simulink model "trackOnly"  (R2014a)
settings: Solver=FixedStepDiscrete  StartTime=0.0  StopTime=10.0  RelTol=1e-3
undefined symbols (not defined in the file or in its folder): fdesignblkfcn, gcbh
libraries: simulink x8, visionstatistics x5, visiontextngfix x2, embdlinuxlib x2
settings Model: SimulationMode=external  ExtModeTrigDuration=100  Creator=jsustare  LastModifiedBy=jsustare
settings OptimizationCC: OptimizeModelRefInitCode=on  LifeSpan=1
settings DebuggingCC: UnderspecifiedInitializationDetection=Classic  SolverPrmCheckMsg=none
settings HardwareCC: ProdLargestAtomicInteger=Long  ProdLargestAtomicFloat=Double  ProdEndianess=LittleEndian  ProdHWDeviceType=ARM Compatible->ARM Cortex
settings RTWCC: SystemTargetFile=realtime.tlc  GenerateMakefile=off  TemplateMakefile=realtime.tmf  Description=Run on Target Hardware  RTWVerbose=off  ProcessScript=realtime_make_rtw_hook
settings STFCustomTargetCC: TargetLibSuffix=.a  GenerateSampleERTMain=on  ConcurrentExecutionCompliant=off  GeneratePreprocessorConditionals=Use local settings  ERTCustomFileBanners=on  SupportNonInlinedSFcns=off  SupportVariableSizeSignals=on  MATLABClassNameForMDSCustomization=Simulink.SoftwareTarget.ERTCustomization  GRTInterface=off  SystemTargetFile=realtime.tlc
settings ERTTargetCC: CombineOutputUpdateFcns=off  SupportContinuousTime=on  SupportVariableSizeSignals=on  ExtModeMexArgs='169.254.0.31' 0 17725  ERTSrcFileBannerTemplate=realtime_code_template.cgt  ERTHdrFileBannerTemplate=realtime_code_template.cgt  ERTDataSrcFileTemplate=realtime_code_template.cgt  ERTDataHdrFileTemplate=realtime_code_template.cgt  ERTCustomFileTemplate=realtime_file_process.tlc

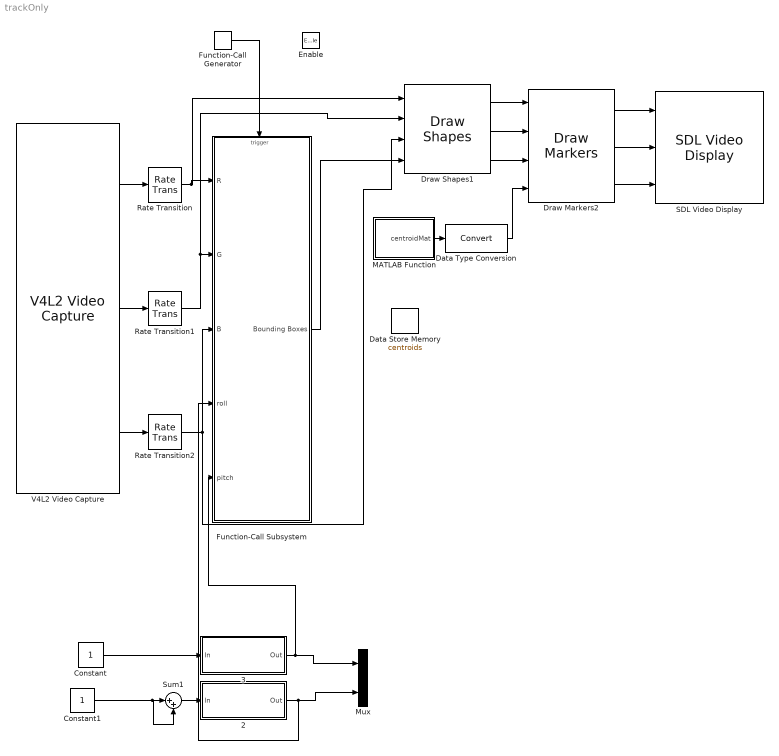
== system trackOnly ==
  Enable : EnablePort  PropagateVarSize=During execution
  " 2" : Subsystem  DialogController=fdesignblkfcn  InitFcn=fdesignblkfcn(gcbh, {'InitFcn'});  mask(Lowpass Filter){}
      mask help: Design a lowpass filter
      settings: CopyFcn=fdesignblkfcn(gcbh, {'CopyFcn'});
      mask Help: helpview(mapfilelocation('dsp'), 'dsplowpassfilter');
      mask Display: disp('Lowpass')
  " 3" : Subsystem  DialogController=fdesignblkfcn  InitFcn=fdesignblkfcn(gcbh, {'InitFcn'});  mask(Lowpass Filter){}
      mask help: Design a lowpass filter
      settings: CopyFcn=fdesignblkfcn(gcbh, {'CopyFcn'});
      mask Help: helpview(mapfilelocation('dsp'), 'dsplowpassfilter');
      mask Display: disp('Lowpass')
  Constant : Constant
  Constant1 : Constant
  Data Store Memory : DataStoreMemory  DataStoreName=centroids  ReadBeforeWriteMsg=warning  WriteAfterWriteMsg=warning  WriteAfterReadMsg=warning  InitialValue=zeros(13,2,4)  OutDataTypeStr=double
  Data Type Conversion : DataTypeConversion
  Draw Markers2 : visiontextngfix/Draw Markers  shape=X-mark  size=3  fill=off  fillClrSource=Specify via dialog  display=User-specified value  intensity=200  color=[255 255 255]  opacity=0.6  viewport=Entire image  antialiasing=off  inType=Obsolete  imagePorts=Separate color signals  prodOutputMode=Binary point scaling  prodOutputWordLength=32  prodOutputFracLength=14  memoryMode=Specify word length  memoryWordLength=16  memoryFracLength=15  roundingMode=Floor  overflowMode=off
  Draw Shapes1 : visiontextngfix/Draw Shapes  shape=Rectangles  fill=off  lineWidth=1  fillClrSource=Specify via dialog  display=User-specified value  intensity=200  color=[255 0 0]  opacity=0.6  viewport=Entire image  antialiasing=off  inType=Obsolete  imagePorts=Separate color signals  prodOutputMode=Binary point scaling  prodOutputWordLength=32  prodOutputFracLength=14  memoryMode=Specify word length  memoryWordLength=16  memoryFracLength=15  roundingMode=Floor  overflowMode=off
  Function-Call Generator : simulink/Ports & Subsystems/Function-Call Generator  sample_time=0.06  numberOfIterations=1
  Function-Call Subsystem : Subsystem  TreatAsAtomicUnit=on
  MATLAB Function : MATLAB Function  TreatAsAtomicUnit=on
  Mux : Mux  Inputs=2
  Rate Transition : RateTransition  Deterministic=off
  Rate Transition1 : RateTransition  Deterministic=off
  Rate Transition2 : RateTransition  Deterministic=off
  SDL Video Display : embdlinuxlib/SDL Video Display  pixelFormat=RGB  pixelOrder=Planar  rowMajor=on  blockPlatform=Raspberry Pi
  Sum1 : Sum  Inputs=|++
  V4L2 Video Capture : embdlinuxlib/V4L2 Video Capture  m_devName='/dev/video0'  roi=[0, 0, 640, 480]  imSizeSelection=320x240  imSize=[640, 480]  pixelFormat=RGB  pixelOrder=Planar  sampleTime=0.06  simOutput=Colorbars  blockPlatform=Raspberry Pi
  wires:
  V4L2 Video Capture/3 -> Rate Transition2/1
  V4L2 Video Capture/1 -> Rate Transition/1
  V4L2 Video Capture/2 -> Rate Transition1/1
  Function-Call Generator/1 -> Function-Call Subsystem/Trigger
  Function-Call Subsystem/1("Bounding Boxes ") -> Draw Shapes1/4
  Rate Transition/1 -> Draw Shapes1/1, Function-Call Subsystem/1(R)
  Rate Transition1/1 -> Draw Shapes1/2, Function-Call Subsystem/2(G)
  Rate Transition2/1 -> Draw Shapes1/3, Function-Call Subsystem/3(B)
  Data Type Conversion/1 -> Draw Markers2/4
  Draw Markers2/2 -> SDL Video Display/2
  Draw Markers2/3 -> SDL Video Display/3
  Draw Markers2/1 -> SDL Video Display/1
  Draw Shapes1/3 -> Draw Markers2/3
  Draw Shapes1/2 -> Draw Markers2/2
  Draw Shapes1/1 -> Draw Markers2/1
  " 2"/1(Out) -> Function-Call Subsystem/4(roll), Mux/2
  " 3"/1(Out) -> Function-Call Subsystem/5(pitch), Mux/1
  Sum1/1 -> " 2"/1(In)
  MATLAB Function/1(centroidMat) -> Data Type Conversion/1
  Constant/1 -> " 3"/1(In)
  Constant1/1 -> Sum1/2, Sum1/1

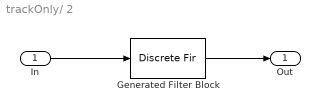
== system trackOnly/ 2 ==
  In : Inport
  Generated Filter Block : DiscreteFir  Tag=BlockMethodSubSystem  Coefficients=[0.0032276888738420255 -0.012093185057654832 -0.056871256727662273 -0.033025317279675399 0.16717851315296134 0.40566714821275895 0.40566714821275895 0.16717851315296134 -0.033025317279675399 -0.056871256727662273 -0.012093185057654832 0.0032276888738420255]  InputProcessing=Columns as channels (frame based)
  Out : Outport
  wires:
  Generated Filter Block/1 -> Out/1
  In/1 -> Generated Filter Block/1

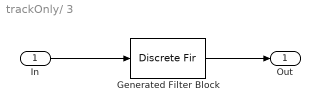
== system trackOnly/ 3 ==
  In : Inport
  Generated Filter Block : DiscreteFir  Tag=BlockMethodSubSystem  Coefficients=[0.0032276888738420255 -0.012093185057654832 -0.056871256727662273 -0.033025317279675399 0.16717851315296134 0.40566714821275895 0.40566714821275895 0.16717851315296134 -0.033025317279675399 -0.056871256727662273 -0.012093185057654832 0.0032276888738420255]  InputProcessing=Columns as channels (frame based)
  Out : Outport
  wires:
  In/1 -> Generated Filter Block/1
  Generated Filter Block/1 -> Out/1

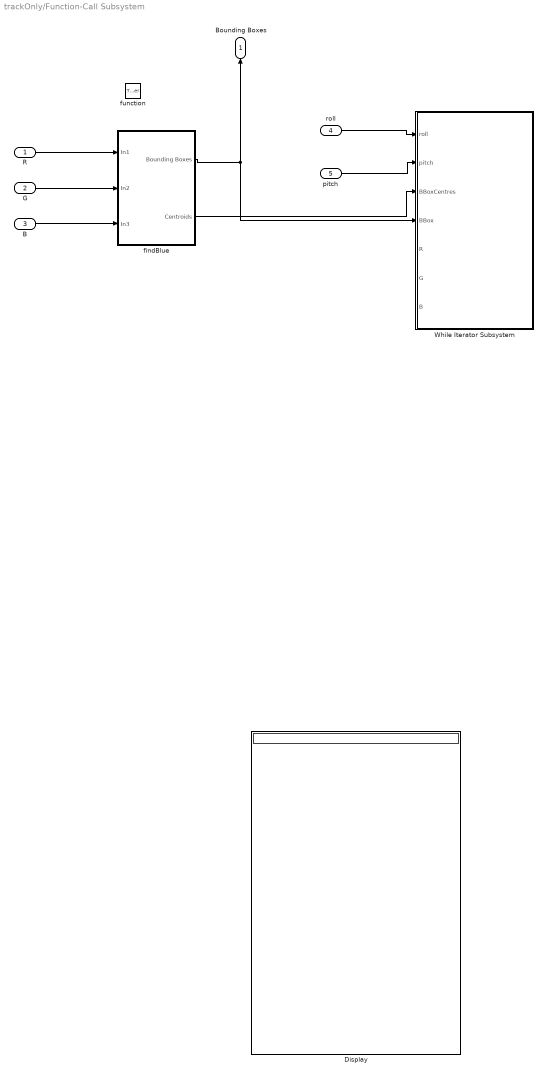
== system trackOnly/Function-Call Subsystem ==
  R : Inport
  G : Inport  Port=2
  B : Inport  Port=3
  roll : Inport  Port=4
  pitch : Inport  Port=5
  function : TriggerPort  TriggerType=function-call
  Display : Display
  While Iterator Subsystem : Subsystem  TreatAsAtomicUnit=on
  findBlue : Subsystem
  "Bounding Boxes " : Outport
  wires:
  G/1 -> findBlue/2(In2)
  R/1 -> findBlue/1(In1)
  B/1 -> findBlue/3(In3)
  findBlue/1(Bounding Boxes) -> While Iterator Subsystem/4(BBox), "Bounding Boxes "/1
  findBlue/2(Centroids) -> While Iterator Subsystem/3(BBoxCentres)
  roll/1 -> While Iterator Subsystem/1(roll)
  pitch/1 -> While Iterator Subsystem/2(pitch)

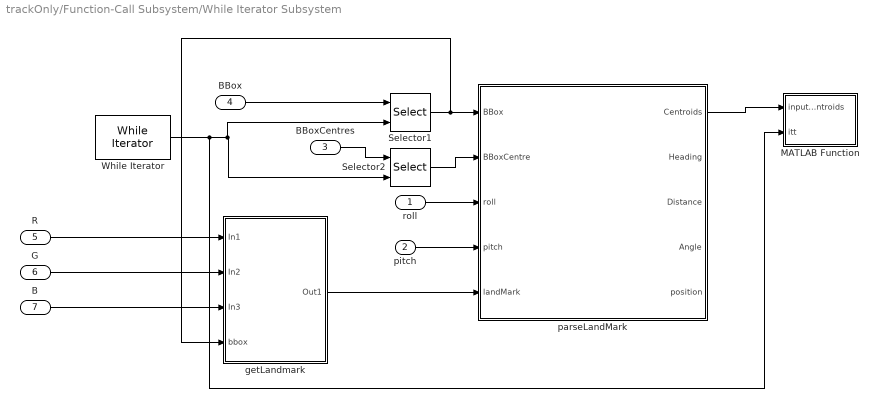
== system trackOnly/Function-Call Subsystem/While Iterator Subsystem ==
  roll : Inport
  pitch : Inport  Port=2
  BBoxCentres : Inport  Port=3
  BBox : Inport  Port=4
  R : Inport  Port=5
  G : Inport  Port=6
  B : Inport  Port=7
  MATLAB Function : MATLAB Function  TreatAsAtomicUnit=on
  Selector1 : Selector  NumberOfDimensions=2  InputPortWidth=3  IndexOptions=Index vector (port),Select all  Indices=[1 3],1  OutputSizes=1,1
  Selector2 : Selector  NumberOfDimensions=2  InputPortWidth=3  IndexOptions=Index vector (port),Select all  Indices=[1 3],1  OutputSizes=1,1
  While Iterator : WhileIterator  MaxIters=4  WhileBlockType=do-while  ShowIterationPort=on
  getLandmark : Subsystem
  parseLandMark : Subsystem
  wires:
  roll/1 -> parseLandMark/3(roll)
  pitch/1 -> parseLandMark/4(pitch)
  While Iterator/1 -> MATLAB Function/2(itt), Selector1/2, Selector2/2
  BBox/1 -> Selector1/1
  BBoxCentres/1 -> Selector2/1
  Selector1/1 -> getLandmark/4(bbox), parseLandMark/1(BBox)
  Selector2/1 -> parseLandMark/2(BBoxCentre)
  R/1 -> getLandmark/1(In1)
  G/1 -> getLandmark/2(In2)
  B/1 -> getLandmark/3(In3)
  getLandmark/1(Out1) -> parseLandMark/5(landMark)
  parseLandMark/1(Centroids) -> MATLAB Function/1(inputCentroids)

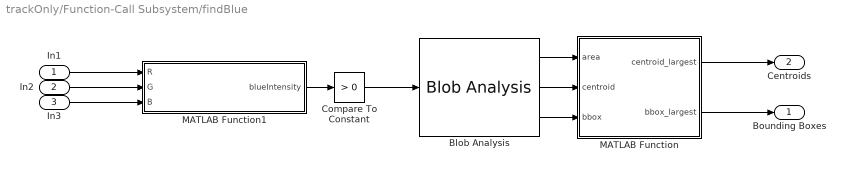
== system trackOnly/Function-Call Subsystem/findBlue ==
  In1 : Inport
  In2 : Inport  Port=2
  In3 : Inport  Port=3
  Blob Analysis : visionstatistics/Blob Analysis  Tag=vipblks_row_conv  area=on  centroid=on  bBox=on  majorAxis=off  minorAxis=off  angle=off  eccentricity=off  equivDiameterSq=off  extent=off  perimeter=off  maxBlobs=16  warnIfNumBlobsExceeded=on  isCount=off  useMinArea=on  minArea=128  useMaxArea=off  maxArea=intmax('uint32')  excludeBorderBlob=on  outDT=double  isOutVarDim=off  isFill=on  fillValues=-1  conn=8  isLabel=off  outputMode=Binary point scaling  outputWordLength=32  outputFracLength=16  firstCoeffMode=Binary point scaling  firstCoeffWordLength=16  firstCoeffFracLength=14  secondCoeffMode=Binary point scaling  secondCoeffWordLength=32  secondCoeffFracLength=16  accumMode=Binary point scaling  accumWordLength=32  accumFracLength=0  prodOutputMode=Binary point scaling  prodOutputWordLength=32  prodOutputFracLength=16  roundingMode=Floor  overflowMode=off
  Compare To Constant : simulink/Logic and Bit Operations/Compare To Constant  relop=>  const=0  OutDataTypeStr=boolean
  MATLAB Function : MATLAB Function  TreatAsAtomicUnit=on
  MATLAB Function1 : MATLAB Function  TreatAsAtomicUnit=on
  Bounding Boxes : Outport
  Centroids : Outport  Port=2
  wires:
  Compare To Constant/1 -> Blob Analysis/1
  Blob Analysis/3 -> MATLAB Function/3(bbox)
  Blob Analysis/1 -> MATLAB Function/1(area)
  MATLAB Function/2(bbox_largest) -> Bounding Boxes/1
  MATLAB Function/1(centroid_largest) -> Centroids/1
  Blob Analysis/2 -> MATLAB Function/2(centroid)
  MATLAB Function1/1(blueIntensity) -> Compare To Constant/1
  In1/1 -> MATLAB Function1/1(R)
  In2/1 -> MATLAB Function1/2(G)
  In3/1 -> MATLAB Function1/3(B)

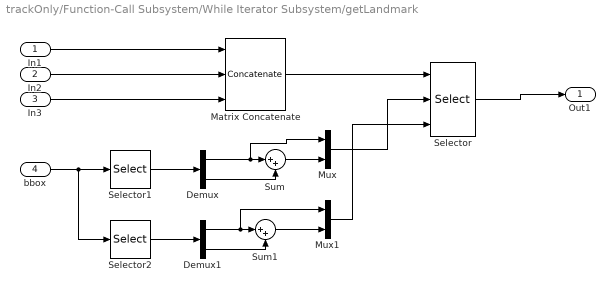
== system trackOnly/Function-Call Subsystem/While Iterator Subsystem/getLandmark ==
  In1 : Inport
  In2 : Inport  Port=2
  In3 : Inport  Port=3
  bbox : Inport  Port=4
  Demux : Demux  Outputs=2
  Demux1 : Demux  Outputs=2
  Matrix Concatenate : Concatenate  NumInputs=3  Mode=Multidimensional array  ConcatenateDimension=3
  Mux : Mux  Inputs=2
  Mux1 : Mux  Inputs=2
  Selector : Selector  NumberOfDimensions=3  InputPortWidth=3  IndexOptions=Starting and ending indices (port),Starting and ending indices (port),Select all  Indices=[1 3],1,1  OutputSizes=1,1,1
  Selector1 : Selector  InputPortWidth=4  Indices=[1 3]
  Selector2 : Selector  InputPortWidth=4  Indices=[2 4]
  Sum : Sum  Inputs=|++
  Sum1 : Sum  Inputs=|++
  Out1 : Outport
  wires:
  In1/1 -> Matrix Concatenate/1
  In2/1 -> Matrix Concatenate/2
  In3/1 -> Matrix Concatenate/3
  Matrix Concatenate/1 -> Selector/1
  bbox/1 -> Selector2/1, Selector1/1
  Selector1/1 -> Demux/1
  Selector2/1 -> Demux1/1
  Demux/1 -> Mux/1, Sum/1
  Demux/2 -> Sum/2
  Demux1/1 -> Mux1/1, Sum1/1
  Demux1/2 -> Sum1/2
  Sum/1 -> Mux/2
  Sum1/1 -> Mux1/2
  Mux/1 -> Selector/2
  Mux1/1 -> Selector/3
  Selector/1 -> Out1/1

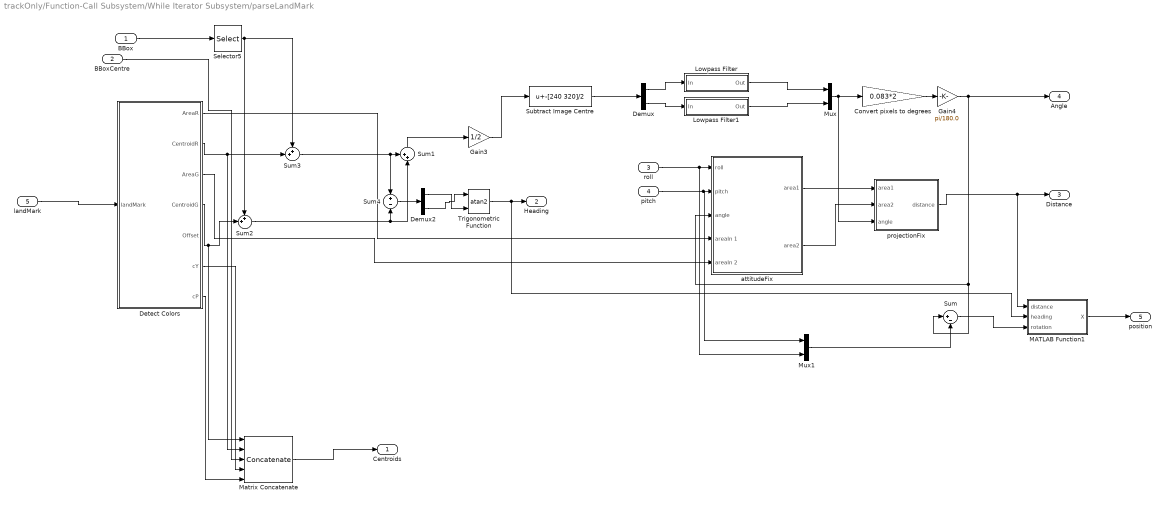
== system trackOnly/Function-Call Subsystem/While Iterator Subsystem/parseLandMark ==
  BBox : Inport
  BBoxCentre : Inport  Port=2
  roll : Inport  Port=3
  pitch : Inport  Port=4
  landMark : Inport  Port=5
  Convert pixels to degrees : Gain  Gain=0.083*2
  Demux : Demux  Outputs=2
  Demux2 : Demux  Outputs=2
  Detect Colors : Subsystem
  Gain3 : Gain  Gain=1/2
  Gain4 : Gain  Gain=pi/180.0
  Lowpass Filter : Subsystem  DialogController=fdesignblkfcn  InitFcn=fdesignblkfcn(gcbh, {'InitFcn'});  mask(Lowpass Filter){}
      mask help: Design a lowpass filter
      settings: CopyFcn=fdesignblkfcn(gcbh, {'CopyFcn'});
      mask Help: helpview(mapfilelocation('dsp'), 'dsplowpassfilter');
      mask Display: disp('Lowpass')
  Lowpass Filter1 : Subsystem  DialogController=fdesignblkfcn  InitFcn=fdesignblkfcn(gcbh, {'InitFcn'});  mask(Lowpass Filter){}
      mask help: Design a lowpass filter
      settings: CopyFcn=fdesignblkfcn(gcbh, {'CopyFcn'});
      mask Help: helpview(mapfilelocation('dsp'), 'dsplowpassfilter');
      mask Display: disp('Lowpass')
  MATLAB Function1 : MATLAB Function  TreatAsAtomicUnit=on
  Matrix Concatenate : Concatenate  NumInputs=5  Mode=Multidimensional array
  Mux : Mux  Inputs=2
  Mux1 : Mux  Inputs=2
  Selector5 : Selector  InputPortWidth=4  Indices=[1 2]
  Subtract Image Centre : Bias  Bias=-[240 320]/2
  Sum : Sum  Inputs=|+-
  Sum1 : Sum  Inputs=++|
  Sum2 : Sum  Inputs=++|
  Sum3 : Sum  Inputs=++|
  Sum4 : Sum  Inputs=+-
  Trigonometric Function : Trigonometry  Operator=atan2
  attitudeFix : Subsystem
  projectionFix : Subsystem
  Centroids : Outport
  Heading : Outport  Port=2
  "Distance " : Outport  Port=3
  Angle : Outport  Port=4
  position : Outport  Port=5
  wires:
  pitch/1 -> Mux1/1, attitudeFix/2(pitch)
  Mux/1 -> projectionFix/3(angle), Convert pixels to degrees/1
  attitudeFix/1(area1) -> projectionFix/1(area1)
  attitudeFix/2(area2) -> projectionFix/2(area2)
  Demux/2 -> Lowpass Filter1/1(In)
  Demux/1 -> Lowpass Filter/1(In)
  Lowpass Filter/1(Out) -> Mux/1
  Lowpass Filter1/1(Out) -> Mux/2
  Selector5/1 -> Sum3/1, Sum2/1
  Sum4/1 -> Demux2/1
  Demux2/2 -> Trigonometric Function/1
  Demux2/1 -> Trigonometric Function/2
  Detect Colors/2(CentroidR) -> Sum3/2, Matrix Concatenate/2
  Sum1/1 -> Gain3/1
  Gain3/1 -> Subtract Image Centre/1
  Sum3/1 -> Sum1/1, Sum4/1
  Subtract Image Centre/1 -> Demux/1
  Convert pixels to degrees/1 -> Gain4/1
  Gain4/1 -> Angle/1, Sum/1, attitudeFix/3("angle ")
  Matrix Concatenate/1 -> Centroids/1
  BBoxCentre/1 -> Matrix Concatenate/3
  Detect Colors/1(AreaR) -> attitudeFix/4(areaIn 1)
  projectionFix/1(distance) -> MATLAB Function1/1(distance), "Distance "/1
  BBox/1 -> Selector5/1
  Detect Colors/4(CentroidG) -> Matrix Concatenate/1, Sum2/2
  Sum2/1 -> Sum1/2, Sum4/2
  Detect Colors/3(AreaG) -> attitudeFix/5(areaIn 2)
  Detect Colors/6(cY) -> Matrix Concatenate/4
  Detect Colors/7(cP) -> Matrix Concatenate/5
  landMark/1 -> Detect Colors/1(landMark)
  Sum/1 -> MATLAB Function1/3(rotation)
  Mux1/1 -> Sum/2
  roll/1 -> Mux1/2, attitudeFix/1(roll)
  Trigonometric Function/1 -> MATLAB Function1/2(heading), Heading/1
  MATLAB Function1/1(X) -> position/1

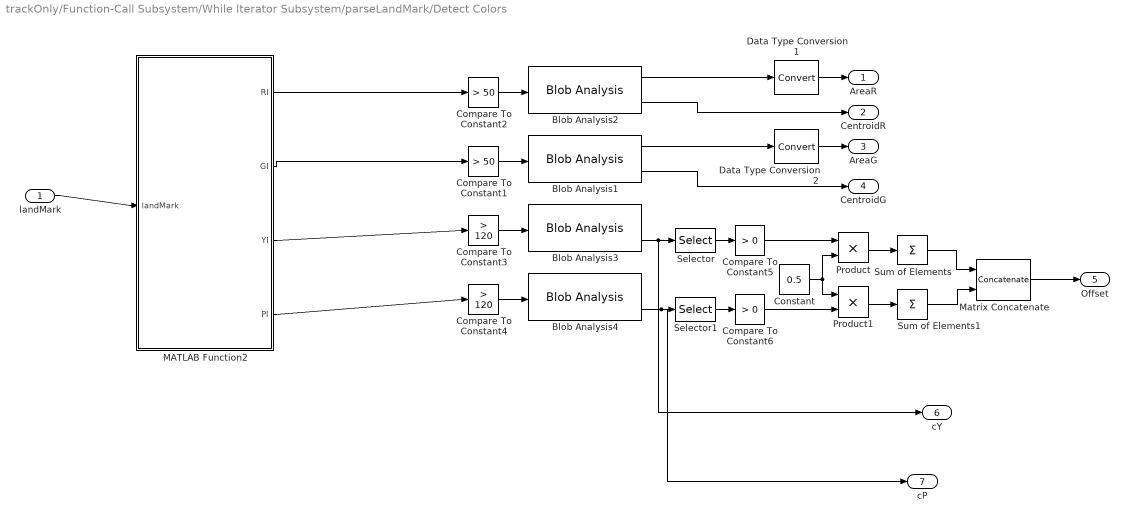
== system trackOnly/Function-Call Subsystem/While Iterator Subsystem/parseLandMark/Detect Colors ==
  landMark : Inport
  Blob Analysis1 : visionstatistics/Blob Analysis  Tag=vipblks_row_conv  area=on  centroid=on  bBox=off  majorAxis=off  minorAxis=off  angle=off  eccentricity=off  equivDiameterSq=off  extent=off  perimeter=off  maxBlobs=1  warnIfNumBlobsExceeded=on  isCount=off  useMinArea=off  minArea=0  useMaxArea=off  maxArea=intmax('uint32')  excludeBorderBlob=off  outDT=double  isOutVarDim=off  isFill=on  fillValues=-1  conn=8  isLabel=off  outputMode=Binary point scaling  outputWordLength=32  outputFracLength=16  firstCoeffMode=Binary point scaling  firstCoeffWordLength=16  firstCoeffFracLength=14  secondCoeffMode=Binary point scaling  secondCoeffWordLength=32  secondCoeffFracLength=16  accumMode=Binary point scaling  accumWordLength=32  accumFracLength=0  prodOutputMode=Binary point scaling  prodOutputWordLength=32  prodOutputFracLength=16  roundingMode=Floor  overflowMode=off
  Blob Analysis2 : visionstatistics/Blob Analysis  Tag=vipblks_row_conv  area=on  centroid=on  bBox=off  majorAxis=off  minorAxis=off  angle=off  eccentricity=off  equivDiameterSq=off  extent=off  perimeter=off  maxBlobs=1  warnIfNumBlobsExceeded=on  isCount=off  useMinArea=off  minArea=0  useMaxArea=off  maxArea=intmax('uint32')  excludeBorderBlob=off  outDT=double  isOutVarDim=off  isFill=on  fillValues=-1  conn=8  isLabel=off  outputMode=Binary point scaling  outputWordLength=32  outputFracLength=16  firstCoeffMode=Binary point scaling  firstCoeffWordLength=16  firstCoeffFracLength=14  secondCoeffMode=Binary point scaling  secondCoeffWordLength=32  secondCoeffFracLength=16  accumMode=Binary point scaling  accumWordLength=32  accumFracLength=0  prodOutputMode=Binary point scaling  prodOutputWordLength=32  prodOutputFracLength=16  roundingMode=Floor  overflowMode=off
  Blob Analysis3 : visionstatistics/Blob Analysis  Tag=vipblks_row_conv  area=on  centroid=on  bBox=off  majorAxis=off  minorAxis=off  angle=off  eccentricity=off  equivDiameterSq=off  extent=off  perimeter=off  maxBlobs=5  warnIfNumBlobsExceeded=on  isCount=off  useMinArea=on  minArea=5  useMaxArea=off  maxArea=intmax('uint32')  excludeBorderBlob=off  outDT=double  isOutVarDim=off  isFill=on  fillValues=-1  conn=8  isLabel=off  outputMode=Binary point scaling  outputWordLength=32  outputFracLength=16  firstCoeffMode=Binary point scaling  firstCoeffWordLength=16  firstCoeffFracLength=14  secondCoeffMode=Binary point scaling  secondCoeffWordLength=32  secondCoeffFracLength=16  accumMode=Binary point scaling  accumWordLength=32  accumFracLength=0  prodOutputMode=Binary point scaling  prodOutputWordLength=32  prodOutputFracLength=16  roundingMode=Floor  overflowMode=off
  Blob Analysis4 : visionstatistics/Blob Analysis  Tag=vipblks_row_conv  area=on  centroid=on  bBox=off  majorAxis=off  minorAxis=off  angle=off  eccentricity=off  equivDiameterSq=off  extent=off  perimeter=off  maxBlobs=5  warnIfNumBlobsExceeded=on  isCount=off  useMinArea=on  minArea=5  useMaxArea=off  maxArea=intmax('uint32')  excludeBorderBlob=off  outDT=double  isOutVarDim=off  isFill=on  fillValues=-1  conn=8  isLabel=off  outputMode=Binary point scaling  outputWordLength=32  outputFracLength=16  firstCoeffMode=Binary point scaling  firstCoeffWordLength=16  firstCoeffFracLength=14  secondCoeffMode=Binary point scaling  secondCoeffWordLength=32  secondCoeffFracLength=16  accumMode=Binary point scaling  accumWordLength=32  accumFracLength=0  prodOutputMode=Binary point scaling  prodOutputWordLength=32  prodOutputFracLength=16  roundingMode=Floor  overflowMode=off
  Compare To Constant1 : simulink/Logic and Bit Operations/Compare To Constant  relop=>  const=50  OutDataTypeStr=boolean
  Compare To Constant2 : simulink/Logic and Bit Operations/Compare To Constant  relop=>  const=50  OutDataTypeStr=boolean
  Compare To Constant3 : simulink/Logic and Bit Operations/Compare To Constant  relop=>  const=120  OutDataTypeStr=boolean
  Compare To Constant4 : simulink/Logic and Bit Operations/Compare To Constant  relop=>  const=120  OutDataTypeStr=boolean
  Compare To Constant5 : simulink/Logic and Bit Operations/Compare To Constant  relop=>  const=0  OutDataTypeStr=boolean
  Compare To Constant6 : simulink/Logic and Bit Operations/Compare To Constant  relop=>  const=0  OutDataTypeStr=boolean
  Constant : Constant  Value=0.5
  Data Type Conversion1 : DataTypeConversion
  Data Type Conversion2 : DataTypeConversion
  MATLAB Function2 : MATLAB Function  TreatAsAtomicUnit=on
  Matrix Concatenate : Concatenate  Mode=Multidimensional array  ConcatenateDimension=2
  Product : Product
  Product1 : Product
  Selector : Selector  NumberOfDimensions=2  InputPortWidth=3  IndexOptions=Select all,Index vector (dialog)  Indices=1,1  OutputSizes=1,1
  Selector1 : Selector  NumberOfDimensions=2  InputPortWidth=3  IndexOptions=Select all,Index vector (dialog)  Indices=1,1  OutputSizes=1,1
  Sum of Elements : Sum  Inputs=+
  Sum of Elements1 : Sum  Inputs=+
  AreaR : Outport
  CentroidR : Outport  Port=2
  AreaG : Outport  Port=3
  CentroidG : Outport  Port=4
  Offset : Outport  Port=5
  cY : Outport  Port=6
  cP : Outport  Port=7
  wires:
  landMark/1 -> MATLAB Function2/1(landMark)
  MATLAB Function2/1(RI) -> Compare To Constant2/1
  Compare To Constant2/1 -> Blob Analysis2/1
  Blob Analysis2/2 -> CentroidR/1
  Blob Analysis2/1 -> Data Type Conversion1/1
  Data Type Conversion1/1 -> AreaR/1
  Compare To Constant1/1 -> Blob Analysis1/1
  Blob Analysis1/2 -> CentroidG/1
  Blob Analysis1/1 -> Data Type Conversion2/1
  Data Type Conversion2/1 -> AreaG/1
  MATLAB Function2/2(GI) -> Compare To Constant1/1
  Compare To Constant3/1 -> Blob Analysis3/1
  MATLAB Function2/3(YI) -> Compare To Constant3/1
  Compare To Constant4/1 -> Blob Analysis4/1
  MATLAB Function2/4(PI) -> Compare To Constant4/1
  Blob Analysis3/2 -> cY/1, Selector/1
  Blob Analysis4/2 -> cP/1, Selector1/1
  Selector/1 -> Compare To Constant5/1
  Selector1/1 -> Compare To Constant6/1
  Compare To Constant5/1 -> Product/1
  Compare To Constant6/1 -> Product1/2
  Constant/1 -> Product1/1, Product/2
  Product/1 -> Sum of Elements/1
  Product1/1 -> Sum of Elements1/1
  Sum of Elements/1 -> Matrix Concatenate/1
  Sum of Elements1/1 -> Matrix Concatenate/2
  Matrix Concatenate/1 -> Offset/1

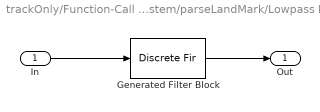
== system trackOnly/Function-Call Subsystem/While Iterator Subsystem/parseLandMark/Lowpass Filter ==
  In : Inport
  Generated Filter Block : DiscreteFir  Tag=BlockMethodSubSystem  Coefficients=[0.0032276888738420255 -0.012093185057654832 -0.056871256727662273 -0.033025317279675399 0.16717851315296134 0.40566714821275895 0.40566714821275895 0.16717851315296134 -0.033025317279675399 -0.056871256727662273 -0.012093185057654832 0.0032276888738420255]  InputProcessing=Columns as channels (frame based)
  Out : Outport
  wires:
  In/1 -> Generated Filter Block/1
  Generated Filter Block/1 -> Out/1

== system trackOnly/Function-Call Subsystem/While Iterator Subsystem/parseLandMark/Lowpass Filter1 ==
  In : Inport
  Generated Filter Block : DiscreteFir  Tag=BlockMethodSubSystem  Coefficients=[0.0032276888738420255 -0.012093185057654832 -0.056871256727662273 -0.033025317279675399 0.16717851315296134 0.40566714821275895 0.40566714821275895 0.16717851315296134 -0.033025317279675399 -0.056871256727662273 -0.012093185057654832 0.0032276888738420255]  InputProcessing=Columns as channels (frame based)
  Out : Outport
  wires:
  Generated Filter Block/1 -> Out/1
  In/1 -> Generated Filter Block/1

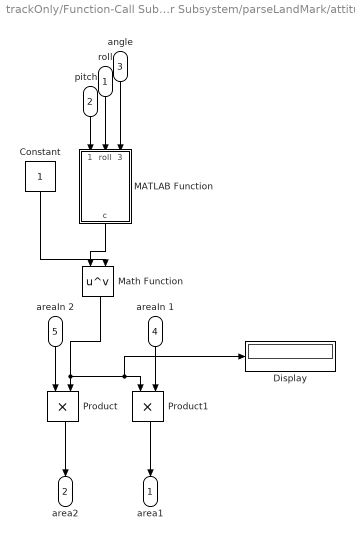
== system trackOnly/Function-Call Subsystem/While Iterator Subsystem/parseLandMark/attitudeFix ==
  roll : Inport
  pitch : Inport  Port=2
  "angle " : Inport  Port=3
  areaIn 1 : Inport  Port=4
  areaIn 2 : Inport  Port=5
  Constant : Constant
  Display : Display
  MATLAB Function : MATLAB Function  TreatAsAtomicUnit=on
  Math Function : Math  Operator=pow  SaturateOnIntegerOverflow=on
  Product : Product
  Product1 : Product
  area1 : Outport
  area2 : Outport  Port=2
  wires:
  pitch/1 -> MATLAB Function/1(pitch)
  roll/1 -> MATLAB Function/2(roll)
  "angle "/1 -> MATLAB Function/3(angle)
  Product1/1 -> area1/1
  Product/1 -> area2/1
  areaIn 2/1 -> Product/1
  areaIn 1/1 -> Product1/2
  MATLAB Function/1(c) -> Math Function/1
  Constant/1 -> Math Function/2
  Math Function/1 -> Display/1, Product1/1, Product/2

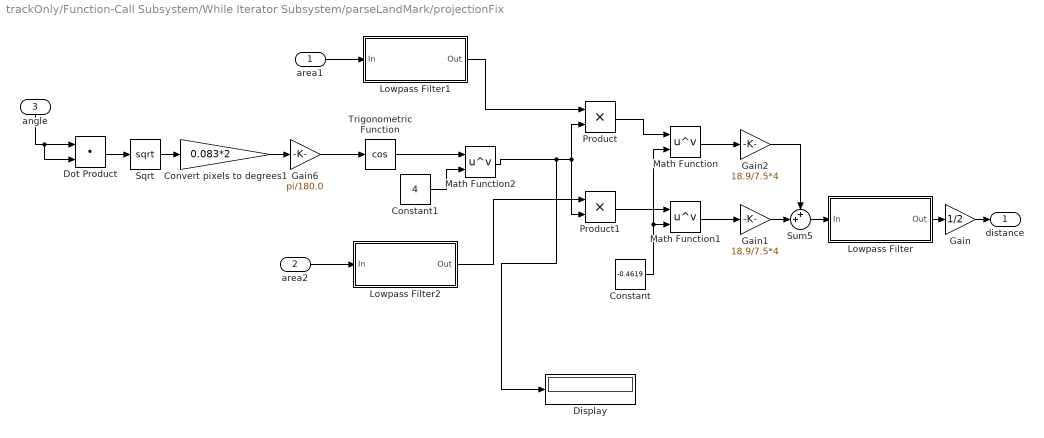
== system trackOnly/Function-Call Subsystem/While Iterator Subsystem/parseLandMark/projectionFix ==
  area1 : Inport
  area2 : Inport  Port=2
  angle : Inport  Port=3
  Constant : Constant  Value=-0.4619
  Constant1 : Constant  Value=4
  Convert pixels to degrees1 : Gain  Gain=0.083*2
  Display : Display
  Dot Product : DotProduct  InputSameDT=on  OutDataTypeStr=Inherit: Inherit via internal rule
  Gain : Gain  Gain=1/2
  Gain1 : Gain  Gain=18.9/7.5*4
  Gain2 : Gain  Gain=18.9/7.5*4
  Gain6 : Gain  Gain=pi/180.0
  Lowpass Filter : Subsystem  DialogController=fdesignblkfcn  InitFcn=fdesignblkfcn(gcbh, {'InitFcn'});  mask(Lowpass Filter){}
      mask help: Design a lowpass filter
      settings: CopyFcn=fdesignblkfcn(gcbh, {'CopyFcn'});
      mask Help: helpview(mapfilelocation('dsp'), 'dsplowpassfilter');
      mask Display: disp('Lowpass')
  Lowpass Filter1 : Subsystem  DialogController=fdesignblkfcn  InitFcn=fdesignblkfcn(gcbh, {'InitFcn'});  mask(Lowpass Filter){}
      mask help: Design a lowpass filter
      settings: CopyFcn=fdesignblkfcn(gcbh, {'CopyFcn'});
      mask Help: helpview(mapfilelocation('dsp'), 'dsplowpassfilter');
      mask Display: disp('Lowpass')
  Lowpass Filter2 : Subsystem  DialogController=fdesignblkfcn  InitFcn=fdesignblkfcn(gcbh, {'InitFcn'});  mask(Lowpass Filter){}
      mask help: Design a lowpass filter
      settings: CopyFcn=fdesignblkfcn(gcbh, {'CopyFcn'});
      mask Help: helpview(mapfilelocation('dsp'), 'dsplowpassfilter');
      mask Display: disp('Lowpass')
  Math Function : Math  Operator=pow  SaturateOnIntegerOverflow=on
  Math Function1 : Math  Operator=pow  SaturateOnIntegerOverflow=on
  Math Function2 : Math  Operator=pow  SaturateOnIntegerOverflow=on
  Product : Product
  Product1 : Product
  Sqrt : Sqrt  SaturateOnIntegerOverflow=on
  Sum5 : Sum  Inputs=++|
  Trigonometric Function : Trigonometry  Operator=cos
  distance : Outport
  wires:
  angle/1 -> Dot Product/2, Dot Product/1
  Math Function1/1 -> Gain1/1
  Math Function/1 -> Gain2/1
  Constant/1 -> Math Function/2, Math Function1/2
  area1/1 -> Lowpass Filter1/1(In)
  area2/1 -> Lowpass Filter2/1(In)
  Gain/1 -> distance/1
  Gain2/1 -> Sum5/1
  Gain1/1 -> Sum5/2
  Lowpass Filter/1(Out) -> Gain/1
  Convert pixels to degrees1/1 -> Gain6/1
  Gain6/1 -> Trigonometric Function/1
  Dot Product/1 -> Sqrt/1
  Sqrt/1 -> Convert pixels to degrees1/1
  Sum5/1 -> Lowpass Filter/1(In)
  Product/1 -> Math Function/1
  Product1/1 -> Math Function1/1
  Math Function2/1 -> Display/1, Product/2, Product1/2
  Trigonometric Function/1 -> Math Function2/1
  Lowpass Filter1/1(Out) -> Product/1
  Lowpass Filter2/1(Out) -> Product1/1
  Constant1/1 -> Math Function2/2

== system trackOnly/Function-Call Subsystem/While Iterator Subsystem/parseLandMark/projectionFix/Lowpass Filter ==
  In : Inport
  Generated Filter Block : DiscreteFir  Tag=BlockMethodSubSystem  Coefficients=[0.011901508381575016 0.02908797826733928 0.0025913585662860131 -0.068996275507793012 -0.050025679925086837 0.16540100530640869 0.41332778671981452 0.41332778671981452 0.16540100530640869 -0.050025679925086837 -0.068996275507793012 0.0025913585662860131 0.02908797826733928 0.011901508381575016]  InputProcessing=Columns as channels (frame based)
  Out : Outport
  wires:
  In/1 -> Generated Filter Block/1
  Generated Filter Block/1 -> Out/1

== system trackOnly/Function-Call Subsystem/While Iterator Subsystem/parseLandMark/projectionFix/Lowpass Filter1 ==
  In : Inport
  Generated Filter Block : DiscreteFir  Tag=BlockMethodSubSystem  Coefficients=[0.011901508381575016 0.02908797826733928 0.0025913585662860131 -0.068996275507793012 -0.050025679925086837 0.16540100530640869 0.41332778671981452 0.41332778671981452 0.16540100530640869 -0.050025679925086837 -0.068996275507793012 0.0025913585662860131 0.02908797826733928 0.011901508381575016]  InputProcessing=Columns as channels (frame based)
  Out : Outport
  wires:
  Generated Filter Block/1 -> Out/1
  In/1 -> Generated Filter Block/1

== system trackOnly/Function-Call Subsystem/While Iterator Subsystem/parseLandMark/projectionFix/Lowpass Filter2 ==
  In : Inport
  Generated Filter Block : DiscreteFir  Tag=BlockMethodSubSystem  Coefficients=[0.011901508381575016 0.02908797826733928 0.0025913585662860131 -0.068996275507793012 -0.050025679925086837 0.16540100530640869 0.41332778671981452 0.41332778671981452 0.16540100530640869 -0.050025679925086837 -0.068996275507793012 0.0025913585662860131 0.02908797826733928 0.011901508381575016]  InputProcessing=Columns as channels (frame based)
  Out : Outport
  wires:
  In/1 -> Generated Filter Block/1
  Generated Filter Block/1 -> Out/1

== matlab function trackOnly/Function-Call Subsystem/While Iterator Subsystem/MATLAB Function ==
  data: inputCentroids input; centroids data_store_memory; itt input
function fcn(inputCentroids, itt)
global centroids;
centroids(:,:,itt)=inputCentroids;

== matlab function trackOnly/Function-Call Subsystem/findBlue/MATLAB Function1 ==
  data: R input; blueIntensity output; G input; B input
function blueIntensity  = fcn(R,G,B)
%#codegen

blueIntensity = B - R - G;

== matlab function trackOnly/Function-Call Subsystem/findBlue/MATLAB Function ==
  data: centroid_largest output; area input; centroid input; bbox_largest output; bbox input
function [centroid_largest, bbox_largest] = selectLargest(area, centroid, bbox)
[y, i] = sort(area);
l=length(area);
bbox_largest = [bbox(i(l),:); bbox(i(l-1),:) ;bbox(i(l-2),:);bbox(i(l-3),:) ];
centroid_largest = [centroid(i(l),:); centroid(i(l-1),:) ;centroid(i(l-2),:);centroid(i(l-3),:) ];

== matlab function trackOnly/MATLAB Function ==
  data: centroidMat output; centroids data_store_memory
function centroidMat = fcn
global centroids;
centroidMat=zeros(13*4,2);
centroidMat(1:13,:)= centroids(:,:,1);
centroidMat(14:26,:)= centroids(:,:,1);
centroidMat(27:39,:)= centroids(:,:,1);
centroidMat(40:52,:)= centroids(:,:,1);

== matlab function trackOnly/Function-Call Subsystem/While Iterator Subsystem/parseLandMark/Detect Colors/MATLAB Function2 ==
  data: landMark input; RI output; GI output; YI output; PI output
function [RI, GI,YI,PI] = fcn(landMark)
RI = landMark(:,:,1) - landMark(:,:,2) - landMark(:,:,3);
GI = landMark(:,:,2) - landMark(:,:,1) - landMark(:,:,3);
YI = landMark(:,:,1) + landMark(:,:,2) - 3*landMark(:,:,3);
PI = landMark(:,:,1) - landMark(:,:,3) - 3*landMark(:,:,2);

== matlab function trackOnly/Function-Call Subsystem/While Iterator Subsystem/parseLandMark/MATLAB Function1 ==
  data: distance input; X output; heading input; rotation input
function X  = fcn(distance,heading,rotation)
X_local = -distance*[sin(rotation(1)); -sin(rotation(2))];
R = [cos(-heading) sin(-heading); -sin(-heading) cos(-heading)];
X = [R*X_local;distance;heading];

== matlab function trackOnly/Function-Call Subsystem/While Iterator Subsystem/parseLandMark/attitudeFix/MATLAB Function ==
  data: pitch input; c output; roll input; angle input
function c = fcn(pitch,roll,angle)
alfa=sqrt((pitch-angle(1))^2 +(roll-angle(2))^2);
c=1/cos(alfa);
